simulink model "ffcontroller"  (R2021a)
settings: Solver=ode4  StartTime=0.0  StopTime=40  FixedStep=1e-3  RelTol=1e-3
settings Model: Creator=brandon  LastModifiedBy=brandon

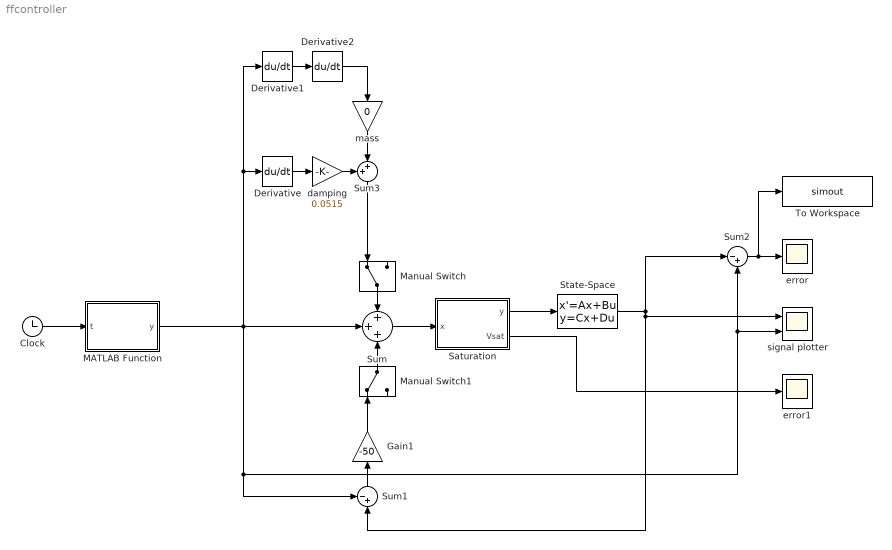
== system ffcontroller ==
  Clock : Clock
  Derivative : Derivative
  Derivative1 : Derivative
  Derivative2 : Derivative
  Gain1 : Gain  Gain=-50
  MATLAB Function : MATLAB Function  TreatAsAtomicUnit=on
  Manual Switch : ManualSwitch
  Manual Switch1 : ManualSwitch
  Saturation : MATLAB Function  TreatAsAtomicUnit=on
  State-Space : StateSpace  A=-19.34  C=20.34  D=0  InitialCondition=5
  Sum : Sum  Inputs=+++
  Sum1 : Sum  Inputs=-+|
  Sum2 : Sum  Inputs=|-+
  Sum3 : Sum  Inputs=++|
  To Workspace : ToWorkspace  VariableName=simout  SaveFormat=Timeseries  SampleTime=-1
  damping : Gain  Gain=0.0515
  error : Scope
  error1 : Scope
  mass : Gain  Gain=0
  signal plotter : Scope  NumInputPorts=2
  wires:
  Clock/1 -> MATLAB Function/1(t)
  MATLAB Function/1(y) -> Sum1/1, Sum2/2, signal plotter/2, Sum/2, Derivative1/1, Derivative/1
  Sum/1 -> Saturation/1(x)
  State-Space/1 -> Sum1/2, signal plotter/1, Sum2/1
  Derivative/1 -> damping/1
  Sum1/1 -> Gain1/1
  Manual Switch/1 -> Sum/1
  Manual Switch1/1 -> Sum/3
  Gain1/1 -> Manual Switch1/1
  Sum2/1 -> error/1, To Workspace/1
  Derivative1/1 -> Derivative2/1
  damping/1 -> Sum3/1
  Sum3/1 -> Manual Switch/1
  mass/1 -> Sum3/2
  Derivative2/1 -> mass/1
  Saturation/1(y) -> State-Space/1
  Saturation/2(Vsat) -> error1/1

== matlab function ffcontroller/MATLAB Function ==
  data: t input; y output
function y = fcn(t)
y = 100*(0.5+0.4*sin(0.25*t^2));

== matlab function ffcontroller/Saturation ==
  data: x input; y output; Vsat output
function [y, Vsat] = fcn(x)
V    = (x+100)/20;        % pressure to voltage
Vsat = min(max(V,0),10);   % bound voltage from 0 to 10v
y    = 100*((Vsat-5)/5);  % convert back to pressure 
end
